simulink model "model_5"  (R2021b)
settings: Solver=VariableStepAuto  StartTime=0.0  StopTime=10  RelTol=1e-3
values from neighbouring files (symbols this model uses):
  A = [-6, -25, -35, -10; 0, -9, -15, 0; 0, 6, 9, 0; 4, 17, 26, 6]    [task_1.m]    (also in task_2.m; task_3.m; task_4.m)
  B = [16, 0; 3, 0; -3, 0; -11, 0]    [task_1.m]    (also in task_2.m; task_3.m = [0; 0; 0; 0]; task_4.m)
  C = eye(4)    [task_1.m]    (also in task_2.m; task_3.m = [2, 2, 0, 4; 0, 3, 6, 0]; task_4.m = [2, 2, 0, 4; 0, 3, 6, 0])
  D = zeros(4, 2)    [task_1.m]    (also in task_2.m; task_3.m = zeros(2, 1); task_4.m = [0, 0; 0, 4])
  K = -inv(R_1)*B'*P_1    [task_4.m]
  L = -P*C'*inv(R)    [task_3.m]    (also in task_4.m)
  Q_1 = 0.1*eye(4)    [task_1.m]    (also in task_2.m = 0.5*eye(4); task_3.m = inv(eye(4)); task_4.m = eye(4))
  R_1 = 10*eye(2)    [task_1.m]    (also in task_2.m = 0.5*eye(2); task_3.m = inv(10*eye(2)); task_4.m = eye(2))
  x0 = [1000; -1000; 1000; -1000]    [task_1.m]    (also in task_2.m; task_3.m = [10; -10; 5; -5]; task_4.m = [10; -10; 5; -5])
  x_0 = [5; 10; -5; 10]    [task_3.m]    (also in task_4.m)
libraries: matrix_library x8
settings Model: Creator=vital  LastModifiedBy=vital

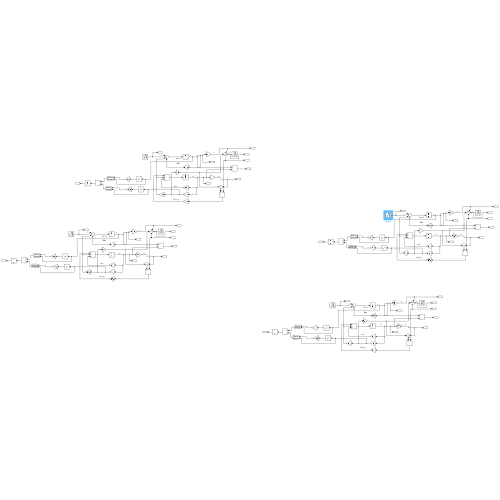
[thumbnail: Simulink's stored preview of the top-level diagram]
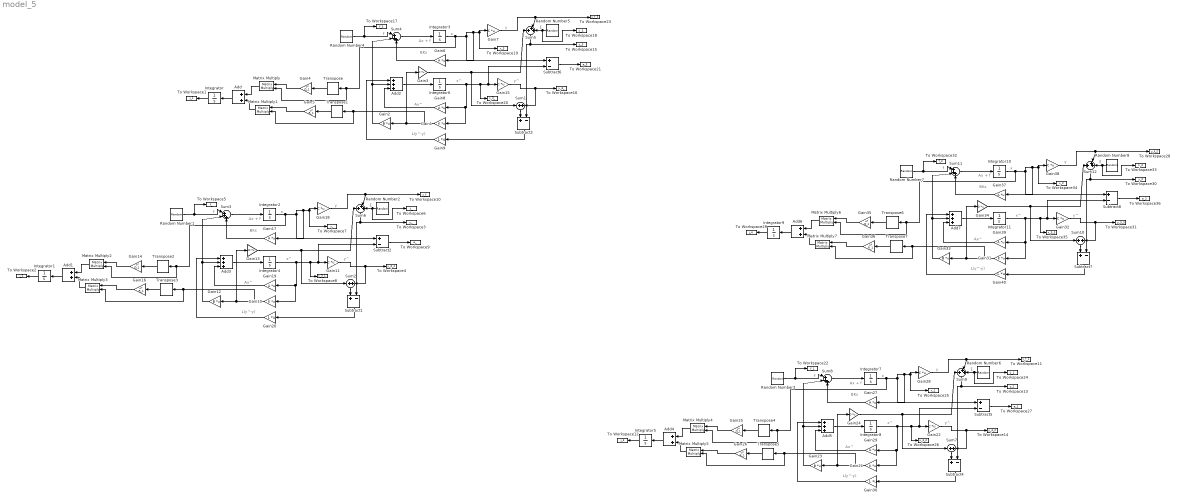
== system model_5 ==
  note: Ax + f
  note: f
  note: x
  note: BKx
  note: Ax^
  note: L(y^-y)
  note: x^
  note: ξ
  note: y^
  note: y
  note: y
  note: y^
  note: ξ
  note: x^
  note: L(y^-y)
  note: BKx
  note: Ax^
  note: x
  note: f
  note: Ax + f
  note: BKx
  note: x
  note: y
  note: ξ
  note: Ax^
  note: x^
  note: f
  note: y^
  note: Ax + f
  note: L(y^-y)
  note: BKx
  note: x
  note: y
  note: ξ
  note: Ax^
  note: x^
  note: f
  note: y^
  note: Ax + f
  note: L(y^-y)
  Add{,1,4,6} (4 alike) : Sum
  Add{2..3,5,7} (4 alike) : Sum  Inputs=+++
  Gain{1,10,21,31} (4 alike) : Gain  Gain=K  Multiplication=Matrix(K*u) (u vector)
  Gain{7,11,15,18,22,28,32,38} (8 alike) : Gain  Gain=C  Multiplication=Matrix(K*u)
  Gain{2,12,23,33} (4 alike) : Gain  Gain=B  Multiplication=Matrix(K*u)
  Gain{3,13,24,34} (4 alike) : Gain  Gain=D  Multiplication=Matrix(K*u) (u vector)
  Gain{4,14,25,35} (4 alike) : Gain  Gain=Q_1  Multiplication=Matrix(u*K)
  Gain{5,16,26,36} (4 alike) : Gain  Gain=R_1  Multiplication=Matrix(u*K)
  Gain{6,17,27,37} (4 alike) : Gain  Gain=A  Multiplication=Matrix(K*u) (u vector)
  Gain{8,19,29,39} (4 alike) : Gain  Gain=A  Multiplication=Matrix(K*u)
  Gain{9,20,30,40} (4 alike) : Gain  Gain=L  Multiplication=Matrix(K*u)
  Integrator{,1,5,9} (4 alike) : Integrator
  Integrator{2..3,7,10} (4 alike) : Integrator  InitialCondition=x0
  Integrator{4,6,8,11} (4 alike) : Integrator  InitialCondition=x_0
  Matrix Multiply{,1..7} (8 alike) : Product  Multiplication=Matrix(*)
  Random Number1 : RandomNumber  Variance=5  Seed=[10; 20; 30; 40]  SampleTime=0000.1
  Random Number2 : RandomNumber  Variance=25  Seed=[50; 60]  SampleTime=0000.1
  Random Number3 : RandomNumber  Variance=5  Seed=[100; 200; 300; 400]  SampleTime=0000.1
  Random Number4 : RandomNumber  Variance=5  Seed=[1; 2; 3; 4]  SampleTime=0000.1
  Random Number5 : RandomNumber  Variance=25  Seed=[5; 6]  SampleTime=0000.1
  Random Number6 : RandomNumber  Variance=25  Seed=[150; 160]  SampleTime=0000.1
  Random Number7 : RandomNumber  Variance=5  Seed=[1000; 2000; 3000; 4000]  SampleTime=0000.1
  Random Number8 : RandomNumber  Variance=25  Seed=[5000; 6000]  SampleTime=0000.1
  Subtract{1..8} (8 alike) : Sum  Inputs=+-
  Sum{1..2,7,10} (4 alike) : Sum  Inputs=+|+
  Sum{3..4,8,11} (4 alike) : Sum  Inputs=|+++
  Sum{5..6,9,12} (4 alike) : Sum  Inputs=+|++
  To Workspace1 : ToWorkspace  VariableName=j_1  SaveFormat=Timeseries  SampleTime=0.0001
  To Workspace10 : ToWorkspace  VariableName=y_f_  SaveFormat=Timeseries  SampleTime=-1
  To Workspace11 : ToWorkspace  VariableName=y_f_1  SaveFormat=Timeseries  SampleTime=-1
  To Workspace12 : ToWorkspace  VariableName=j_3  SaveFormat=Timeseries  SampleTime=0.0001
  To Workspace13 : ToWorkspace  VariableName=y_1  SaveFormat=Timeseries  SampleTime=-1
  To Workspace14 : ToWorkspace  VariableName=y_3_2  SaveFormat=Timeseries  SampleTime=-1
  To Workspace15 : ToWorkspace  VariableName=y_3  SaveFormat=Timeseries  SampleTime=-1
  To Workspace16 : ToWorkspace  VariableName=y_3_  SaveFormat=Timeseries  SampleTime=-1
  To Workspace17 : ToWorkspace  VariableName=f_3  SaveFormat=Timeseries  SampleTime=-1
  To Workspace18 : ToWorkspace  VariableName=k_3  SaveFormat=Timeseries  SampleTime=-1
  To Workspace19 : ToWorkspace  VariableName=x_3  SaveFormat=Timeseries  SampleTime=0.0001
  To Workspace2 : ToWorkspace  VariableName=j_2  SaveFormat=Timeseries  SampleTime=0.0001
  To Workspace20 : ToWorkspace  VariableName=x_3_  SaveFormat=Timeseries  SampleTime=-1
  To Workspace21 : ToWorkspace  VariableName=e_3  SaveFormat=Timeseries  SampleTime=-1
  To Workspace22 : ToWorkspace  VariableName=f_1  SaveFormat=Timeseries  SampleTime=-1
  To Workspace23 : ToWorkspace  VariableName=y_f_3  SaveFormat=Timeseries  SampleTime=-1
  To Workspace24 : ToWorkspace  VariableName=k_1  SaveFormat=Timeseries  SampleTime=-1
  To Workspace25 : ToWorkspace  VariableName=x_1  SaveFormat=Timeseries  SampleTime=0.0001
  To Workspace26 : ToWorkspace  VariableName=x_3_2  SaveFormat=Timeseries  SampleTime=-1
  To Workspace27 : ToWorkspace  VariableName=e_1  SaveFormat=Timeseries  SampleTime=-1
  To Workspace28 : ToWorkspace  VariableName=y_f_2  SaveFormat=Timeseries  SampleTime=-1
  To Workspace29 : ToWorkspace  VariableName=j_4  SaveFormat=Timeseries  SampleTime=0.0001
  To Workspace3 : ToWorkspace  VariableName=y_  SaveFormat=Timeseries  SampleTime=-1
  To Workspace30 : ToWorkspace  VariableName=y_2  SaveFormat=Timeseries  SampleTime=-1
  To Workspace31 : ToWorkspace  VariableName=y_3_3  SaveFormat=Timeseries  SampleTime=-1
  To Workspace32 : ToWorkspace  VariableName=f_2  SaveFormat=Timeseries  SampleTime=-1
  To Workspace33 : ToWorkspace  VariableName=k_2  SaveFormat=Timeseries  SampleTime=-1
  To Workspace34 : ToWorkspace  VariableName=x_2  SaveFormat=Timeseries  SampleTime=0.0001
  To Workspace35 : ToWorkspace  VariableName=x_3_3  SaveFormat=Timeseries  SampleTime=-1
  To Workspace36 : ToWorkspace  VariableName=e_2  SaveFormat=Timeseries  SampleTime=-1
  To Workspace4 : ToWorkspace  VariableName=y_3_1  SaveFormat=Timeseries  SampleTime=-1
  To Workspace5 : ToWorkspace  VariableName=f_  SaveFormat=Timeseries  SampleTime=-1
  To Workspace6 : ToWorkspace  VariableName=k_  SaveFormat=Timeseries  SampleTime=-1
  To Workspace7 : ToWorkspace  VariableName=x_  SaveFormat=Timeseries  SampleTime=0.0001
  To Workspace8 : ToWorkspace  VariableName=x_3_1  SaveFormat=Timeseries  SampleTime=-1
  To Workspace9 : ToWorkspace  VariableName=e_  SaveFormat=Timeseries  SampleTime=-1
  Transpose{,1..7} (8 alike) : matrix_library/Transpose
      settings: SourceProductBaseCode=SL
  wires:
  Subtract3/1 -> Gain9/1
  Random Number5/1 -> Sum5/3, To Workspace18/1
  Integrator3/1 -> Matrix Multiply/2, Transpose/1, To Workspace19/1, Gain7/1, Gain6/1, Subtract6/1
  Sum5/1 -> To Workspace15/1, Subtract3/2
  Sum4/1 -> Integrator3/1
  Subtract6/1 -> To Workspace21/1
  Random Number4/1 -> Sum4/1, To Workspace17/1
  Gain3/1 -> Sum1/1, Sum5/1
  Gain2/1 -> Sum4/2, Add2/2
  Gain9/1 -> Add2/1
  Gain1/1 -> Transpose1/1, Matrix Multiply1/2, Gain3/1, Gain2/1
  Add2/1 -> Integrator6/1
  Gain7/1 -> Sum5/2, To Workspace23/1
  Gain8/1 -> Add2/3
  Sum1/1 -> Subtract3/1
  Gain6/1 -> Sum4/3
  Gain15/1 -> Sum1/2, To Workspace16/1
  Integrator6/1 -> Gain1/1, Gain8/1, To Workspace20/1, Subtract6/2, Gain15/1
  Transpose1/1 -> Gain5/1
  Transpose/1 -> Gain4/1
  Matrix Multiply/1 -> Add/1
  Matrix Multiply1/1 -> Add/2
  Add/1 -> Integrator/1
  Integrator/1 -> To Workspace1/1
  Gain5/1 -> Matrix Multiply1/1
  Gain4/1 -> Matrix Multiply/1
  Integrator4/1 -> Gain10/1, Gain19/1, To Workspace8/1, Subtract2/2, Gain11/1
  Gain17/1 -> Sum3/3
  Add3/1 -> Integrator4/1
  Gain18/1 -> Sum6/2, To Workspace10/1
  Gain10/1 -> Transpose3/1, Matrix Multiply3/2, Gain13/1, Gain12/1
  Gain19/1 -> Add3/3
  Gain13/1 -> Sum2/1, Sum6/1
  Gain12/1 -> Sum3/2, Add3/2
  Gain20/1 -> Add3/1
  Subtract2/1 -> To Workspace9/1
  Random Number1/1 -> Sum3/1, To Workspace5/1
  Sum3/1 -> Integrator2/1
  Integrator2/1 -> Matrix Multiply2/2, Transpose2/1, To Workspace7/1, Gain18/1, Gain17/1, Subtract2/1
  Gain11/1 -> Sum2/2, To Workspace4/1
  Random Number2/1 -> Sum6/3, To Workspace6/1
  Transpose2/1 -> Gain14/1
  Matrix Multiply2/1 -> Add1/1
  Add1/1 -> Integrator1/1
  Sum6/1 -> To Workspace3/1, Subtract1/2
  Gain16/1 -> Matrix Multiply3/1
  Integrator1/1 -> To Workspace2/1
  Subtract1/1 -> Gain20/1
  Matrix Multiply3/1 -> Add1/2
  Sum2/1 -> Subtract1/1
  Gain14/1 -> Matrix Multiply2/1
  Transpose3/1 -> Gain16/1
  Transpose5/1 -> Gain26/1
  Gain25/1 -> Matrix Multiply4/1
  Sum7/1 -> Subtract4/1
  Integrator5/1 -> To Workspace12/1
  Sum9/1 -> To Workspace13/1, Subtract4/2
  Random Number6/1 -> Sum9/3, To Workspace24/1
  Subtract4/1 -> Gain30/1
  Transpose4/1 -> Gain25/1
  Integrator7/1 -> Matrix Multiply4/2, Transpose4/1, To Workspace25/1, Gain28/1, Gain27/1, Subtract5/1
  Subtract5/1 -> To Workspace27/1
  Gain26/1 -> Matrix Multiply5/1
  Random Number3/1 -> Sum8/1, To Workspace22/1
  Gain22/1 -> Sum7/2, To Workspace14/1
  Sum8/1 -> Integrator7/1
  Gain29/1 -> Add5/3
  Gain23/1 -> Sum8/2, Add5/2
  Gain21/1 -> Transpose5/1, Matrix Multiply5/2, Gain24/1, Gain23/1
  Gain24/1 -> Sum7/1, Sum9/1
  Gain30/1 -> Add5/1
  Gain28/1 -> Sum9/2, To Workspace11/1
  Add5/1 -> Integrator8/1
  Gain27/1 -> Sum8/3
  Integrator8/1 -> Gain21/1, Gain29/1, To Workspace26/1, Subtract5/2, Gain22/1
  Add4/1 -> Integrator5/1
  Matrix Multiply4/1 -> Add4/1
  Matrix Multiply5/1 -> Add4/2
  Transpose7/1 -> Gain36/1
  Gain35/1 -> Matrix Multiply6/1
  Sum10/1 -> Subtract7/1
  Integrator9/1 -> To Workspace29/1
  Sum12/1 -> To Workspace30/1, Subtract7/2
  Random Number8/1 -> Sum12/3, To Workspace33/1
  Subtract7/1 -> Gain40/1
  Transpose6/1 -> Gain35/1
  Integrator10/1 -> Matrix Multiply6/2, Transpose6/1, To Workspace34/1, Gain38/1, Gain37/1, Subtract8/1
  Subtract8/1 -> To Workspace36/1
  Gain36/1 -> Matrix Multiply7/1
  Random Number7/1 -> Sum11/1, To Workspace32/1
  Gain32/1 -> Sum10/2, To Workspace31/1
  Sum11/1 -> Integrator10/1
  Gain39/1 -> Add7/3
  Gain33/1 -> Sum11/2, Add7/2
  Gain31/1 -> Transpose7/1, Matrix Multiply7/2, Gain34/1, Gain33/1
  Gain34/1 -> Sum10/1, Sum12/1
  Gain40/1 -> Add7/1
  Gain38/1 -> Sum12/2, To Workspace28/1
  Add7/1 -> Integrator11/1
  Gain37/1 -> Sum11/3
  Integrator11/1 -> Gain31/1, Gain39/1, To Workspace35/1, Subtract8/2, Gain32/1
  Add6/1 -> Integrator9/1
  Matrix Multiply6/1 -> Add6/1
  Matrix Multiply7/1 -> Add6/2
